simulink model "sim_SS_H2DF_2024a_GRU"  (R2024a)
settings: Solver=FixedStepAuto  StartTime=0.0  StopTime=4899  FixedStep=1  RelTol=1e-3  EnableMultiTasking=on
model workspace (MAT data in the model file):
  enable_IMEP_noise = 100
  enable_IMEP_offset = 1
values from neighbouring files (symbols this model uses):
  C2C_NMPC = init_C2C_NMPC_H2DF(C2C_NMPC.expdata)    [run_SS_H2DF_control.m]
undefined symbols (not defined in the file or in its folder): cost_length, horizon_length, y_ref_buf
libraries: matrix_library x3
(part 2 of 3)

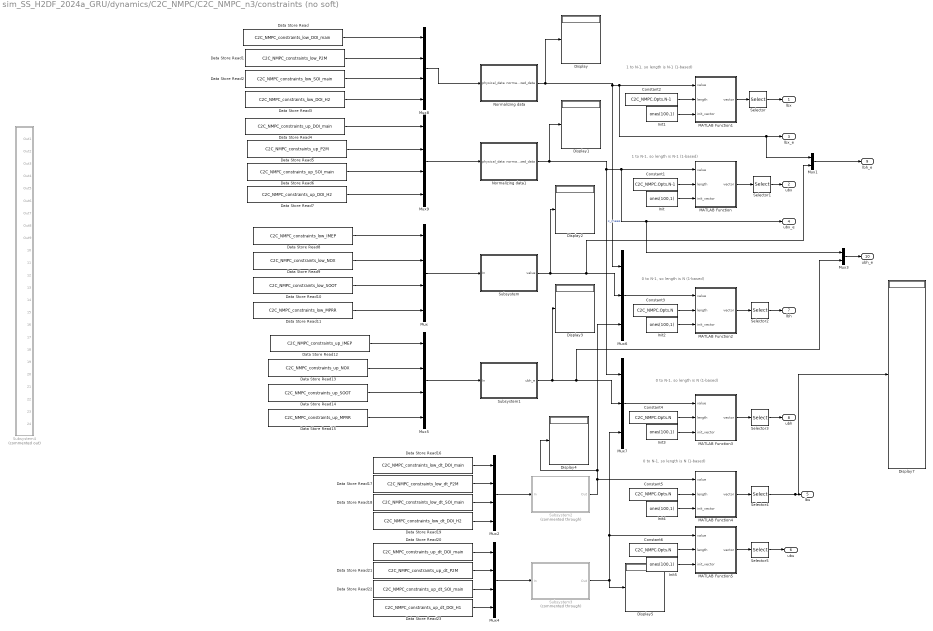
== system sim_SS_H2DF_2024a_GRU/dynamics/C2C_NMPC/C2C_NMPC_n3/constraints (no soft) ==
  note: 1 to N-1, so length is N-1 (1-based)
  note: 1 to N-1, so length is N-1 (1-based)
  note: 0 to N-1, so length is N (1-based)
  note: 0 to N-1, so length is N (1-based)
  note: 0 to N-1, so length is N (1-based)
  Constant1 : Constant  Value=C2C_NMPC.Opts.N-1
  Constant2 : Constant  Value=C2C_NMPC.Opts.N-1
  Constant{3..6} (4 alike) : Constant  Value=C2C_NMPC.Opts.N
  Data Store Read : DataStoreRead  DataStoreName=C2C_NMPC_constraints_low_DOI_main  IndexOptions=Index vector (dialog)  Indices=1  OutputSizes=1
  Data Store Read1 : DataStoreRead  DataStoreName=C2C_NMPC_constraints_low_P2M  IndexOptions=Index vector (dialog)  Indices=1  OutputSizes=1
  Data Store Read10 : DataStoreRead  DataStoreName=C2C_NMPC_constraints_low_SOOT  IndexOptions=Index vector (dialog)  Indices=1  OutputSizes=1
  Data Store Read11 : DataStoreRead  DataStoreName=C2C_NMPC_constraints_low_MPRR  IndexOptions=Index vector (dialog)  Indices=1  OutputSizes=1
  Data Store Read12 : DataStoreRead  DataStoreName=C2C_NMPC_constraints_up_IMEP  IndexOptions=Index vector (dialog)  Indices=1  OutputSizes=1
  Data Store Read13 : DataStoreRead  DataStoreName=C2C_NMPC_constraints_up_NOX  IndexOptions=Index vector (dialog)  Indices=1  OutputSizes=1
  Data Store Read14 : DataStoreRead  DataStoreName=C2C_NMPC_constraints_up_SOOT  IndexOptions=Index vector (dialog)  Indices=1  OutputSizes=1
  Data Store Read15 : DataStoreRead  DataStoreName=C2C_NMPC_constraints_up_MPRR  IndexOptions=Index vector (dialog)  Indices=1  OutputSizes=1
  Data Store Read16 : DataStoreRead  DataStoreName=C2C_NMPC_constraints_low_dt_DOI_main  IndexOptions=Index vector (dialog)  Indices=1  OutputSizes=1
  Data Store Read17 : DataStoreRead  DataStoreName=C2C_NMPC_constraints_low_dt_P2M  IndexOptions=Index vector (dialog)  Indices=1  OutputSizes=1
  Data Store Read18 : DataStoreRead  DataStoreName=C2C_NMPC_constraints_low_dt_SOI_main  IndexOptions=Index vector (dialog)  Indices=1  OutputSizes=1
  Data Store Read19 : DataStoreRead  DataStoreName=C2C_NMPC_constraints_low_dt_DOI_H2  IndexOptions=Index vector (dialog)  Indices=1  OutputSizes=1
  Data Store Read2 : DataStoreRead  DataStoreName=C2C_NMPC_constraints_low_SOI_main  IndexOptions=Index vector (dialog)  Indices=1  OutputSizes=1
  Data Store Read20 : DataStoreRead  DataStoreName=C2C_NMPC_constraints_up_dt_DOI_main  IndexOptions=Index vector (dialog)  Indices=1  OutputSizes=1
  Data Store Read21 : DataStoreRead  DataStoreName=C2C_NMPC_constraints_up_dt_P2M  IndexOptions=Index vector (dialog)  Indices=1  OutputSizes=1
  Data Store Read22 : DataStoreRead  DataStoreName=C2C_NMPC_constraints_up_dt_SOI_main  IndexOptions=Index vector (dialog)  Indices=1  OutputSizes=1
  Data Store Read23 : DataStoreRead  DataStoreName=C2C_NMPC_constraints_up_dt_DOI_H1  IndexOptions=Index vector (dialog)  Indices=1  OutputSizes=1
  Data Store Read3 : DataStoreRead  DataStoreName=C2C_NMPC_constraints_low_DOI_H2  IndexOptions=Index vector (dialog)  Indices=1  OutputSizes=1
  Data Store Read4 : DataStoreRead  DataStoreName=C2C_NMPC_constraints_up_DOI_main  IndexOptions=Index vector (dialog)  Indices=1  OutputSizes=1
  Data Store Read5 : DataStoreRead  DataStoreName=C2C_NMPC_constraints_up_P2M  IndexOptions=Index vector (dialog)  Indices=1  OutputSizes=1
  Data Store Read6 : DataStoreRead  DataStoreName=C2C_NMPC_constraints_up_SOI_main  IndexOptions=Index vector (dialog)  Indices=1  OutputSizes=1
  Data Store Read7 : DataStoreRead  DataStoreName=C2C_NMPC_constraints_up_DOI_H2  IndexOptions=Index vector (dialog)  Indices=1  OutputSizes=1
  Data Store Read8 : DataStoreRead  DataStoreName=C2C_NMPC_constraints_low_IMEP  IndexOptions=Index vector (dialog)  Indices=1  OutputSizes=1
  Data Store Read9 : DataStoreRead  DataStoreName=C2C_NMPC_constraints_low_NOX  IndexOptions=Index vector (dialog)  Indices=1  OutputSizes=1
  Display{,1..5,7} (7 alike) : Display
  Init{,1..5} (6 alike) : Constant  Value=ones(100,1)
  MATLAB Function : MATLAB Function  TreatAsAtomicUnit=on
  MATLAB Function1 : MATLAB Function  TreatAsAtomicUnit=on
  MATLAB Function2 : MATLAB Function  TreatAsAtomicUnit=on
  MATLAB Function3 : MATLAB Function  TreatAsAtomicUnit=on
  MATLAB Function4 : MATLAB Function  TreatAsAtomicUnit=on
  MATLAB Function5 : MATLAB Function  TreatAsAtomicUnit=on
  Mux{,2,4..5,8..9} (6 alike) : Mux
  Mux1 : Mux  Inputs=2
  Mux3 : Mux  Inputs=2
  Mux6 : Mux  Inputs=3
  Mux7 : Mux  Inputs=3
  Normalizing data : Subsystem
  Normalizing data1 : Subsystem
  Selector : Selector  IndexOptions=Index vector (dialog)  Indices=1:((C2C_NMPC.Opts.N-1)*C2C_NMPC.Dims.n_controls)  OutputSizes=1
  Selector1 : Selector  IndexOptions=Index vector (dialog)  Indices=1:((C2C_NMPC.Opts.N-1)*C2C_NMPC.Dims.n_controls)  OutputSizes=1
  Selector2 : Selector  IndexOptions=Index vector (dialog)  Indices=1:((C2C_NMPC.Opts.N)*(C2C_NMPC.Dims.n_outputs + C2C_NMPC.Dims.n_controls +C2C_NMPC.Dims.n_controls))  OutputSizes=1
  Selector3 : Selector  IndexOptions=Index vector (dialog)  Indices=1:((C2C_NMPC.Opts.N)*(C2C_NMPC.Dims.n_outputs + C2C_NMPC.Dims.n_controls +C2C_NMPC.Dims.n_controls))  OutputSizes=1
  Selector4 : Selector  IndexOptions=Index vector (dialog)  Indices=1:((C2C_NMPC.Opts.N)*(C2C_NMPC.Dims.n_controls))  OutputSizes=1
  Selector5 : Selector  IndexOptions=Index vector (dialog)  Indices=1:((C2C_NMPC.Opts.N)*(C2C_NMPC.Dims.n_controls))  OutputSizes=1
  Subsystem : Subsystem
  Subsystem1 : Subsystem
  Subsystem2 : Subsystem  Commented=through
  Subsystem3 : Subsystem  Commented=through
  Subsystem4 : Subsystem  Commented=on
  lbx : Outport
  ubx : Outport  Port=2
  lbx_e : Outport  Port=3
  ubx_e : Outport  Port=4
  lbu : Outport  Port=5
  ubu : Outport  Port=6
  lbh : Outport  Port=7
  ubh : Outport  Port=8
  lbh_e : Outport  Port=9
  ubh_e : Outport  Port=10
  wires:
  Selector4/1 -> lbu/1, Display7/1
  Selector5/1 -> ubu/1
  Constant6/1 -> MATLAB Function5/2(length)
  Init5/1 -> MATLAB Function5/3(init_vector)
  MATLAB Function5/1(vector) -> Selector5/1
  MATLAB Function4/1(vector) -> Selector4/1
  Init4/1 -> MATLAB Function4/3(init_vector)
  Constant5/1 -> MATLAB Function4/2(length)
  Data Store Read23/1 -> Mux4/4
  Data Store Read22/1 -> Mux4/3
  Data Store Read21/1 -> Mux4/2
  Data Store Read20/1 -> Mux4/1
  Data Store Read19/1 -> Mux2/4
  Data Store Read18/1 -> Mux2/3
  Data Store Read17/1 -> Mux2/2
  Data Store Read16/1 -> Mux2/1
  Data Store Read15/1 -> Mux5/4
  Data Store Read14/1 -> Mux5/3
  Data Store Read13/1 -> Mux5/2
  Data Store Read12/1 -> Mux5/1
  Data Store Read11/1 -> Mux/4
  Data Store Read10/1 -> Mux/3
  Data Store Read9/1 -> Mux/2
  Data Store Read8/1 -> Mux/1
  Mux3/1 -> ubh_e/1
  Subsystem1/1(ubh_e) -> Mux7/2, Mux3/2, Display3/1
  Mux1/1 -> lbh_e/1
  Selector3/1 -> ubh/1
  Selector2/1 -> lbh/1
  Selector1/1 -> ubx/1
  Data Store Read7/1 -> Mux9/4
  Normalizing data1/1(normalized_data) -> MATLAB Function/1(value), ubx_e/1, Mux3/1, Mux7/1, Display1/1  "x_meas"
  Mux9/1 -> Normalizing data1/1(physical_data)
  Data Store Read4/1 -> Mux9/1
  Data Store Read5/1 -> Mux9/2
  Data Store Read6/1 -> Mux9/3
  Selector/1 -> lbx/1
  Mux8/1 -> Normalizing data/1(physical_data)
  Data Store Read/1 -> Mux8/1
  Data Store Read1/1 -> Mux8/2
  Data Store Read2/1 -> Mux8/3
  Data Store Read3/1 -> Mux8/4
  Constant4/1 -> MATLAB Function3/2(length)
  Init3/1 -> MATLAB Function3/3(init_vector)
  Mux7/1 -> MATLAB Function3/1(value)
  MATLAB Function3/1(vector) -> Selector3/1
  Subsystem2/1(Out) -> Mux6/3, Display4/1, MATLAB Function4/1(value)
  Subsystem/1(value) -> Mux6/2, Mux1/2, Display2/1
  Normalizing data/1(normalized_data) -> Display/1, MATLAB Function1/1(value), lbx_e/1, Mux1/1, Mux6/1
  Mux6/1 -> MATLAB Function2/1(value)
  Subsystem3/1(Out) -> Display5/1, Mux7/3, MATLAB Function5/1(value)
  Init2/1 -> MATLAB Function2/3(init_vector)
  Constant3/1 -> MATLAB Function2/2(length)
  MATLAB Function2/1(vector) -> Selector2/1
  Init1/1 -> MATLAB Function1/3(init_vector)
  Constant2/1 -> MATLAB Function1/2(length)
  MATLAB Function1/1(vector) -> Selector/1
  MATLAB Function/1(vector) -> Selector1/1
  Constant1/1 -> MATLAB Function/2(length)
  Init/1 -> MATLAB Function/3(init_vector)
  Mux4/1 -> Subsystem3/1(In)
  Mux2/1 -> Subsystem2/1(In)
  Mux5/1 -> Subsystem1/1(In)
  Mux/1 -> Subsystem/1(In)

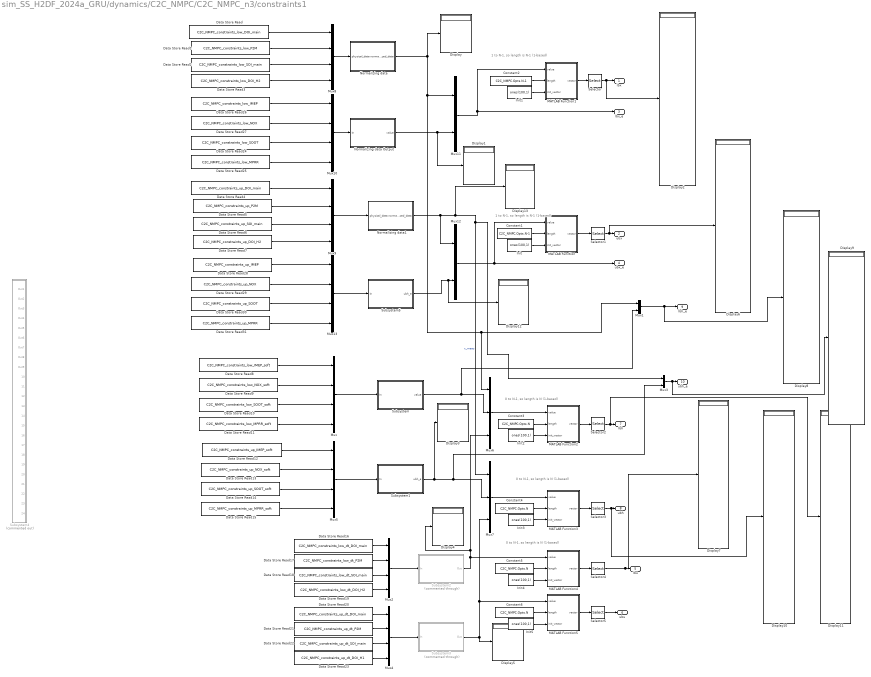
== system sim_SS_H2DF_2024a_GRU/dynamics/C2C_NMPC/C2C_NMPC_n3/constraints1 ==
  note: 0 to N-1, so length is N (1-based)
  note: 0 to N-1, so length is N (1-based)
  note: 0 to N-1, so length is N (1-based)
  note: 1 to N-1, so length is N-1 (1-based)
  note: 1 to N-1, so length is N-1 (1-based)
  Constant1 : Constant  Value=C2C_NMPC.Opts.N-1
  Constant2 : Constant  Value=C2C_NMPC.Opts.N-1
  Constant{3..6} (4 alike) : Constant  Value=C2C_NMPC.Opts.N
  Data Store Read : DataStoreRead  DataStoreName=C2C_NMPC_constraints_low_DOI_main  IndexOptions=Index vector (dialog)  Indices=1  OutputSizes=1
  Data Store Read1 : DataStoreRead  DataStoreName=C2C_NMPC_constraints_low_P2M  IndexOptions=Index vector (dialog)  Indices=1  OutputSizes=1
  Data Store Read10 : DataStoreRead  DataStoreName=C2C_NMPC_constraints_low_SOOT_soft  IndexOptions=Index vector (dialog)  Indices=1  OutputSizes=1
  Data Store Read11 : DataStoreRead  DataStoreName=C2C_NMPC_constraints_low_MPRR_soft  IndexOptions=Index vector (dialog)  Indices=1  OutputSizes=1
  Data Store Read12 : DataStoreRead  DataStoreName=C2C_NMPC_constraints_up_IMEP_soft  IndexOptions=Index vector (dialog)  Indices=1  OutputSizes=1
  Data Store Read13 : DataStoreRead  DataStoreName=C2C_NMPC_constraints_up_NOX_soft  IndexOptions=Index vector (dialog)  Indices=1  OutputSizes=1
  Data Store Read14 : DataStoreRead  DataStoreName=C2C_NMPC_constraints_up_SOOT_soft  IndexOptions=Index vector (dialog)  Indices=1  OutputSizes=1
  Data Store Read15 : DataStoreRead  DataStoreName=C2C_NMPC_constraints_up_MPRR_soft  IndexOptions=Index vector (dialog)  Indices=1  OutputSizes=1
  Data Store Read16 : DataStoreRead  DataStoreName=C2C_NMPC_constraints_low_dt_DOI_main  IndexOptions=Index vector (dialog)  Indices=1  OutputSizes=1
  Data Store Read17 : DataStoreRead  DataStoreName=C2C_NMPC_constraints_low_dt_P2M  IndexOptions=Index vector (dialog)  Indices=1  OutputSizes=1
  Data Store Read18 : DataStoreRead  DataStoreName=C2C_NMPC_constraints_low_dt_SOI_main  IndexOptions=Index vector (dialog)  Indices=1  OutputSizes=1
  Data Store Read19 : DataStoreRead  DataStoreName=C2C_NMPC_constraints_low_dt_DOI_H2  IndexOptions=Index vector (dialog)  Indices=1  OutputSizes=1
  Data Store Read2 : DataStoreRead  DataStoreName=C2C_NMPC_constraints_low_SOI_main  IndexOptions=Index vector (dialog)  Indices=1  OutputSizes=1
  Data Store Read20 : DataStoreRead  DataStoreName=C2C_NMPC_constraints_up_dt_DOI_main  IndexOptions=Index vector (dialog)  Indices=1  OutputSizes=1
  Data Store Read21 : DataStoreRead  DataStoreName=C2C_NMPC_constraints_up_dt_P2M  IndexOptions=Index vector (dialog)  Indices=1  OutputSizes=1
  Data Store Read22 : DataStoreRead  DataStoreName=C2C_NMPC_constraints_up_dt_SOI_main  IndexOptions=Index vector (dialog)  Indices=1  OutputSizes=1
  Data Store Read23 : DataStoreRead  DataStoreName=C2C_NMPC_constraints_up_dt_DOI_H1  IndexOptions=Index vector (dialog)  Indices=1  OutputSizes=1
  Data Store Read24 : DataStoreRead  DataStoreName=C2C_NMPC_constraints_low_SOOT  IndexOptions=Index vector (dialog)  Indices=1  OutputSizes=1
  Data Store Read25 : DataStoreRead  DataStoreName=C2C_NMPC_constraints_low_MPRR  IndexOptions=Index vector (dialog)  Indices=1  OutputSizes=1
  Data Store Read26 : DataStoreRead  DataStoreName=C2C_NMPC_constraints_low_IMEP  IndexOptions=Index vector (dialog)  Indices=1  OutputSizes=1
  Data Store Read27 : DataStoreRead  DataStoreName=C2C_NMPC_constraints_low_NOX  IndexOptions=Index vector (dialog)  Indices=1  OutputSizes=1
  Data Store Read28 : DataStoreRead  DataStoreName=C2C_NMPC_constraints_up_IMEP  IndexOptions=Index vector (dialog)  Indices=1  OutputSizes=1
  Data Store Read29 : DataStoreRead  DataStoreName=C2C_NMPC_constraints_up_NOX  IndexOptions=Index vector (dialog)  Indices=1  OutputSizes=1
  Data Store Read3 : DataStoreRead  DataStoreName=C2C_NMPC_constraints_low_DOI_H2  IndexOptions=Index vector (dialog)  Indices=1  OutputSizes=1
  Data Store Read30 : DataStoreRead  DataStoreName=C2C_NMPC_constraints_up_SOOT  IndexOptions=Index vector (dialog)  Indices=1  OutputSizes=1
  Data Store Read31 : DataStoreRead  DataStoreName=C2C_NMPC_constraints_up_MPRR  IndexOptions=Index vector (dialog)  Indices=1  OutputSizes=1
  Data Store Read4 : DataStoreRead  DataStoreName=C2C_NMPC_constraints_up_DOI_main  IndexOptions=Index vector (dialog)  Indices=1  OutputSizes=1
  Data Store Read5 : DataStoreRead  DataStoreName=C2C_NMPC_constraints_up_P2M  IndexOptions=Index vector (dialog)  Indices=1  OutputSizes=1
  Data Store Read6 : DataStoreRead  DataStoreName=C2C_NMPC_constraints_up_SOI_main  IndexOptions=Index vector (dialog)  Indices=1  OutputSizes=1
  Data Store Read7 : DataStoreRead  DataStoreName=C2C_NMPC_constraints_up_DOI_H2  IndexOptions=Index vector (dialog)  Indices=1  OutputSizes=1
  Data Store Read8 : DataStoreRead  DataStoreName=C2C_NMPC_constraints_low_IMEP_soft  IndexOptions=Index vector (dialog)  Indices=1  OutputSizes=1
  Data Store Read9 : DataStoreRead  DataStoreName=C2C_NMPC_constraints_low_NOX_soft  IndexOptions=Index vector (dialog)  Indices=1  OutputSizes=1
  Display{,1..13} (14 alike) : Display
  Init{,1..5} (6 alike) : Constant  Value=ones(100,1)
  MATLAB Function : MATLAB Function  TreatAsAtomicUnit=on
  MATLAB Function1 : MATLAB Function  TreatAsAtomicUnit=on
  MATLAB Function2 : MATLAB Function  TreatAsAtomicUnit=on
  MATLAB Function3 : MATLAB Function  TreatAsAtomicUnit=on
  MATLAB Function4 : MATLAB Function  TreatAsAtomicUnit=on
  MATLAB Function5 : MATLAB Function  TreatAsAtomicUnit=on
  Mux{,2,4..5,8..10,13} (8 alike) : Mux
  Mux{1,3,11..12} (4 alike) : Mux  Inputs=2
  Mux6 : Mux  Inputs=3
  Mux7 : Mux  Inputs=3
  Normalizing data : Subsystem
  Normalizing data Output : Subsystem
  Normalizing data1 : Subsystem
  Selector : Selector  IndexOptions=Index vector (dialog)  Indices=1:((C2C_NMPC.Opts.N-1)*(C2C_NMPC.Dims.n_controls+C2C_NMPC.Dims.n_outputs))  OutputSizes=1
  Selector1 : Selector  IndexOptions=Index vector (dialog)  Indices=1:((C2C_NMPC.Opts.N-1)*(C2C_NMPC.Dims.n_controls+C2C_NMPC.Dims.n_outputs))  OutputSizes=1
  Selector2 : Selector  IndexOptions=Index vector (dialog)  Indices=1:((C2C_NMPC.Opts.N-1)*(C2C_NMPC.Dims.n_outputs + C2C_NMPC.Dims.n_controls +C2C_NMPC.Dims.n_controls))  OutputSizes=1
  Selector3 : Selector  IndexOptions=Index vector (dialog)  Indices=1:((C2C_NMPC.Opts.N-1)*(C2C_NMPC.Dims.n_outputs + C2C_NMPC.Dims.n_controls +C2C_NMPC.Dims.n_controls))  OutputSizes=1
  Selector4 : Selector  IndexOptions=Index vector (dialog)  Indices=1:((C2C_NMPC.Opts.N)*(C2C_NMPC.Dims.n_controls))  OutputSizes=1
  Selector5 : Selector  IndexOptions=Index vector (dialog)  Indices=1:((C2C_NMPC.Opts.N)*(C2C_NMPC.Dims.n_controls))  OutputSizes=1
  Subsystem : Subsystem
  Subsystem1 : Subsystem
  Subsystem2 : Subsystem  Commented=through
  Subsystem3 : Subsystem  Commented=through
  Subsystem4 : Subsystem  Commented=on
  Subsystem5 : Subsystem
  lbx : Outport
  ubx : Outport  Port=2
  lbx_e : Outport  Port=3
  ubx_e : Outport  Port=4
  lbu : Outport  Port=5
  ubu : Outport  Port=6
  lbh : Outport  Port=7
  ubh : Outport  Port=8
  lbh_e : Outport  Port=9
  ubh_e : Outport  Port=10
  wires:
  Mux/1 -> Subsystem/1(In)
  Mux5/1 -> Subsystem1/1(In)
  Mux2/1 -> Subsystem2/1(In)
  Mux4/1 -> Subsystem3/1(In)
  Init/1 -> MATLAB Function/3(init_vector)
  Constant1/1 -> MATLAB Function/2(length)
  MATLAB Function/1(vector) -> Selector1/1
  MATLAB Function1/1(vector) -> Selector/1
  Constant2/1 -> MATLAB Function1/2(length)
  Init1/1 -> MATLAB Function1/3(init_vector)
  MATLAB Function2/1(vector) -> Selector2/1
  Constant3/1 -> MATLAB Function2/2(length)
  Init2/1 -> MATLAB Function2/3(init_vector)
  Subsystem3/1(Out) -> MATLAB Function5/1(value), Mux7/3, Display5/1
  Mux6/1 -> MATLAB Function2/1(value)
  Subsystem/1(value) -> Mux1/2, Mux6/2
  Subsystem2/1(Out) -> MATLAB Function4/1(value), Display4/1, Mux6/3
  MATLAB Function3/1(vector) -> Selector3/1
  Mux7/1 -> MATLAB Function3/1(value)
  Init3/1 -> MATLAB Function3/3(init_vector)
  Constant4/1 -> MATLAB Function3/2(length)
  Data Store Read3/1 -> Mux8/4
  Data Store Read2/1 -> Mux8/3
  Data Store Read1/1 -> Mux8/2
  Data Store Read/1 -> Mux8/1
  Mux8/1 -> Normalizing data/1(physical_data)
  Selector/1 -> Display2/1, lbx/1
  Data Store Read6/1 -> Mux9/3
  Data Store Read5/1 -> Mux9/2
  Data Store Read4/1 -> Mux9/1
  Mux9/1 -> Normalizing data1/1(physical_data)
  Normalizing data1/1(normalized_data) -> Mux12/1, Display13/1, Mux7/1, Mux3/1  "x_meas"
  Data Store Read7/1 -> Mux9/4
  Selector1/1 -> Display6/1, ubx/1
  Selector2/1 -> Display11/1, lbh/1
  Selector3/1 -> Display10/1, ubh/1
  Mux1/1 -> Display8/1, lbh_e/1
  Subsystem1/1(ubh_e) -> Display3/1, Mux3/2, Mux7/2
  Mux3/1 -> Display9/1, ubh_e/1
  Data Store Read8/1 -> Mux/1
  Data Store Read9/1 -> Mux/2
  Data Store Read10/1 -> Mux/3
  Data Store Read11/1 -> Mux/4
  Data Store Read12/1 -> Mux5/1
  Data Store Read13/1 -> Mux5/2
  Data Store Read14/1 -> Mux5/3
  Data Store Read15/1 -> Mux5/4
  Data Store Read16/1 -> Mux2/1
  Data Store Read17/1 -> Mux2/2
  Data Store Read18/1 -> Mux2/3
  Data Store Read19/1 -> Mux2/4
  Data Store Read20/1 -> Mux4/1
  Data Store Read21/1 -> Mux4/2
  Data Store Read22/1 -> Mux4/3
  Data Store Read23/1 -> Mux4/4
  Constant5/1 -> MATLAB Function4/2(length)
  Init4/1 -> MATLAB Function4/3(init_vector)
  MATLAB Function4/1(vector) -> Selector4/1
  MATLAB Function5/1(vector) -> Selector5/1
  Init5/1 -> MATLAB Function5/3(init_vector)
  Constant6/1 -> MATLAB Function5/2(length)
  Selector5/1 -> ubu/1
  Selector4/1 -> Display7/1, lbu/1
  Data Store Read27/1 -> Mux10/2
  Data Store Read26/1 -> Mux10/1
  Data Store Read24/1 -> Mux10/3
  Data Store Read25/1 -> Mux10/4
  Mux10/1 -> Normalizing data Output/1(In)
  Mux11/1 -> lbx_e/1, MATLAB Function1/1(value)
  Normalizing data Output/1(value) -> Display1/1, Mux11/2
  Mux12/1 -> MATLAB Function/1(value), ubx_e/1
  Mux13/1 -> Subsystem5/1(In)
  Data Store Read30/1 -> Mux13/3
  Data Store Read29/1 -> Mux13/2
  Data Store Read28/1 -> Mux13/1
  Subsystem5/1(ubh_e) -> Display12/1, Mux12/2
  Data Store Read31/1 -> Mux13/4
  Normalizing data/1(normalized_data) -> Mux6/1, Mux1/1, Mux11/1, Display/1

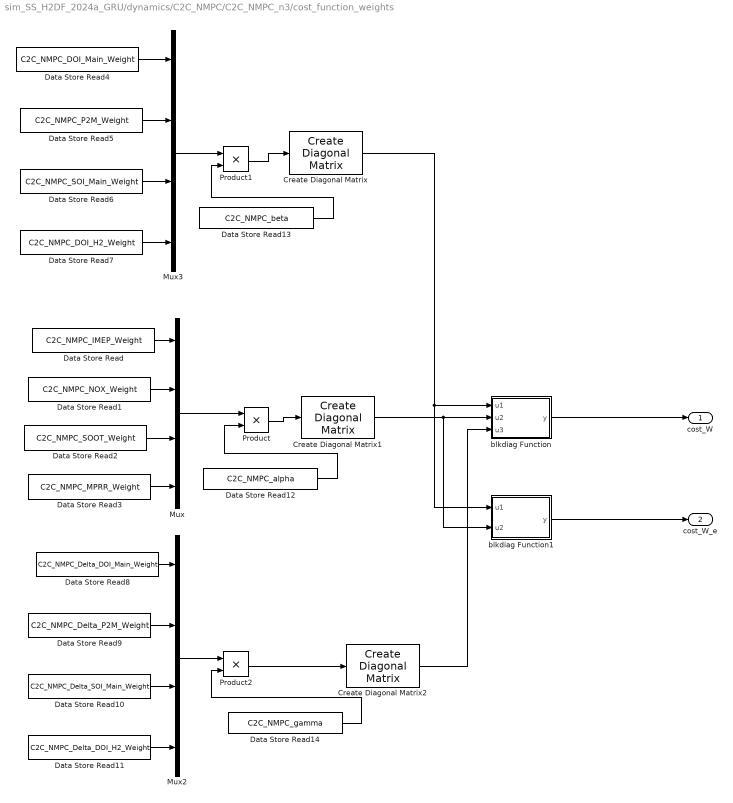
== system sim_SS_H2DF_2024a_GRU/dynamics/C2C_NMPC/C2C_NMPC_n3/cost_function_weights ==
  Create Diagonal Matrix : matrix_library/Create Diagonal Matrix
  Create Diagonal Matrix1 : matrix_library/Create Diagonal Matrix
  Create Diagonal Matrix2 : matrix_library/Create Diagonal Matrix
  Data Store Read : DataStoreRead  DataStoreName=C2C_NMPC_IMEP_Weight  IndexOptions=Index vector (dialog)  Indices=1  OutputSizes=1
  Data Store Read1 : DataStoreRead  DataStoreName=C2C_NMPC_NOX_Weight  IndexOptions=Index vector (dialog)  Indices=1  OutputSizes=1
  Data Store Read10 : DataStoreRead  DataStoreName=C2C_NMPC_Delta_SOI_Main_Weight  IndexOptions=Index vector (dialog)  Indices=1  OutputSizes=1
  Data Store Read11 : DataStoreRead  DataStoreName=C2C_NMPC_Delta_DOI_H2_Weight  IndexOptions=Index vector (dialog)  Indices=1  OutputSizes=1
  Data Store Read12 : DataStoreRead  DataStoreName=C2C_NMPC_alpha  IndexOptions=Index vector (dialog)  Indices=1  OutputSizes=1
  Data Store Read13 : DataStoreRead  DataStoreName=C2C_NMPC_beta  IndexOptions=Index vector (dialog)  Indices=1  OutputSizes=1
  Data Store Read14 : DataStoreRead  DataStoreName=C2C_NMPC_gamma  IndexOptions=Index vector (dialog)  Indices=1  OutputSizes=1
  Data Store Read2 : DataStoreRead  DataStoreName=C2C_NMPC_SOOT_Weight  IndexOptions=Index vector (dialog)  Indices=1  OutputSizes=1
  Data Store Read3 : DataStoreRead  DataStoreName=C2C_NMPC_MPRR_Weight  IndexOptions=Index vector (dialog)  Indices=1  OutputSizes=1
  Data Store Read4 : DataStoreRead  DataStoreName=C2C_NMPC_DOI_Main_Weight  IndexOptions=Index vector (dialog)  Indices=1  OutputSizes=1
  Data Store Read5 : DataStoreRead  DataStoreName=C2C_NMPC_P2M_Weight  IndexOptions=Index vector (dialog)  Indices=1  OutputSizes=1
  Data Store Read6 : DataStoreRead  DataStoreName=C2C_NMPC_SOI_Main_Weight  IndexOptions=Index vector (dialog)  Indices=1  OutputSizes=1
  Data Store Read7 : DataStoreRead  DataStoreName=C2C_NMPC_DOI_H2_Weight  IndexOptions=Index vector (dialog)  Indices=1  OutputSizes=1
  Data Store Read8 : DataStoreRead  DataStoreName=C2C_NMPC_Delta_DOI_Main_Weight  IndexOptions=Index vector (dialog)  Indices=1  OutputSizes=1
  Data Store Read9 : DataStoreRead  DataStoreName=C2C_NMPC_Delta_P2M_Weight  IndexOptions=Index vector (dialog)  Indices=1  OutputSizes=1
  Mux : Mux
  Mux2 : Mux
  Mux3 : Mux
  Product : Product
  Product1 : Product
  Product2 : Product
  blkdiag Function : MATLAB Function  TreatAsAtomicUnit=on
  blkdiag Function1 : MATLAB Function  TreatAsAtomicUnit=on
  cost_W : Outport
  cost_W_e : Outport  Port=2
  wires:
  blkdiag Function1/1(y) -> cost_W_e/1
  Mux2/1 -> Product2/1
  Data Store Read14/1 -> Product2/2
  Data Store Read13/1 -> Product1/2
  Data Store Read12/1 -> Product/2
  Data Store Read11/1 -> Mux2/4
  Data Store Read10/1 -> Mux2/3
  Data Store Read9/1 -> Mux2/2
  Data Store Read8/1 -> Mux2/1
  Create Diagonal Matrix/1 -> blkdiag Function/1(u1), blkdiag Function1/1(u1)
  Data Store Read2/1 -> Mux/3
  Data Store Read3/1 -> Mux/4
  Data Store Read/1 -> Mux/1
  Data Store Read1/1 -> Mux/2
  Mux/1 -> Product/1
  Product/1 -> Create Diagonal Matrix1/1
  Product1/1 -> Create Diagonal Matrix/1
  Mux3/1 -> Product1/1
  Data Store Read5/1 -> Mux3/2
  Data Store Read6/1 -> Mux3/3
  Data Store Read4/1 -> Mux3/1
  Data Store Read7/1 -> Mux3/4
  Create Diagonal Matrix1/1 -> blkdiag Function/2(u2), blkdiag Function1/2(u2)
  Product2/1 -> Create Diagonal Matrix2/1
  Create Diagonal Matrix2/1 -> blkdiag Function/3(u3)
  blkdiag Function/1(y) -> cost_W/1

== system sim_SS_H2DF_2024a_GRU/dynamics/C2C_NMPC/C2C_NMPC_n3/constraints (no soft)/Normalizing data ==
  physical_data : Inport
  Constant1 : Constant  Value=C2C_NMPC.Normalization.controls.mean(2)
  Constant2 : Constant  Value=C2C_NMPC.Normalization.controls.mean(3)
  Constant3 : Constant  Value=C2C_NMPC.Normalization.controls.mean(1)
  Constant4 : Constant  Value=C2C_NMPC.Normalization.controls.mean(4)
  Gain1 : Gain  Gain=1/C2C_NMPC.Normalization.controls.std(2)
  Gain2 : Gain  Gain=1/C2C_NMPC.Normalization.controls.std(3)
  Gain3 : Gain  Gain=1/C2C_NMPC.Normalization.controls.std(4)
  Gain4 : Gain  Gain=1/C2C_NMPC.Normalization.controls.std(1)
  Mux : Mux
  Selector : Selector  IndexOptions=Index vector (dialog)  Indices=[2]  OutputSizes=1
  Selector1 : Selector  IndexOptions=Index vector (dialog)  Indices=[1]  OutputSizes=1
  Selector2 : Selector  IndexOptions=Index vector (dialog)  Indices=[3]  OutputSizes=1
  Selector3 : Selector  IndexOptions=Index vector (dialog)  Indices=[4]  OutputSizes=1
  Sum{1..4} (4 alike) : Sum  Inputs=|+-
  normalized_data : Outport
  wires:
  physical_data/1 -> Selector2/1, Selector3/1, Selector/1, Selector1/1
  Mux/1 -> normalized_data/1
  Gain3/1 -> Mux/4
  Gain2/1 -> Mux/3
  Gain1/1 -> Mux/2
  Gain4/1 -> Mux/1
  Selector1/1 -> Sum4/1
  Selector3/1 -> Sum1/1
  Constant4/1 -> Sum1/2
  Sum1/1 -> Gain3/1
  Sum2/1 -> Gain1/1
  Constant1/1 -> Sum2/2
  Selector/1 -> Sum2/1
  Sum3/1 -> Gain2/1
  Sum4/1 -> Gain4/1
  Constant2/1 -> Sum3/2
  Selector2/1 -> Sum3/1
  Constant3/1 -> Sum4/2

== system sim_SS_H2DF_2024a_GRU/dynamics/C2C_NMPC/C2C_NMPC_n3/constraints (no soft)/Normalizing data1 ==
  physical_data : Inport
  Constant1 : Constant  Value=C2C_NMPC.Normalization.controls.mean(2)
  Constant2 : Constant  Value=C2C_NMPC.Normalization.controls.mean(3)
  Constant3 : Constant  Value=C2C_NMPC.Normalization.controls.mean(1)
  Constant4 : Constant  Value=C2C_NMPC.Normalization.controls.mean(4)
  Gain1 : Gain  Gain=1/C2C_NMPC.Normalization.controls.std(2)
  Gain2 : Gain  Gain=1/C2C_NMPC.Normalization.controls.std(3)
  Gain3 : Gain  Gain=1/C2C_NMPC.Normalization.controls.std(4)
  Gain4 : Gain  Gain=1/C2C_NMPC.Normalization.controls.std(1)
  Mux : Mux
  Selector : Selector  IndexOptions=Index vector (dialog)  Indices=[2]  OutputSizes=1
  Selector1 : Selector  IndexOptions=Index vector (dialog)  Indices=[1]  OutputSizes=1
  Selector2 : Selector  IndexOptions=Index vector (dialog)  Indices=[3]  OutputSizes=1
  Selector3 : Selector  IndexOptions=Index vector (dialog)  Indices=[4]  OutputSizes=1
  Sum{1..4} (4 alike) : Sum  Inputs=|+-
  normalized_data : Outport
  wires:
  physical_data/1 -> Selector2/1, Selector3/1, Selector/1, Selector1/1
  Mux/1 -> normalized_data/1
  Gain3/1 -> Mux/4
  Gain2/1 -> Mux/3
  Gain1/1 -> Mux/2
  Gain4/1 -> Mux/1
  Selector1/1 -> Sum4/1
  Selector3/1 -> Sum1/1
  Constant4/1 -> Sum1/2
  Sum1/1 -> Gain3/1
  Sum2/1 -> Gain1/1
  Constant1/1 -> Sum2/2
  Selector/1 -> Sum2/1
  Sum3/1 -> Gain2/1
  Sum4/1 -> Gain4/1
  Constant2/1 -> Sum3/2
  Selector2/1 -> Sum3/1
  Constant3/1 -> Sum4/2

== system sim_SS_H2DF_2024a_GRU/dynamics/C2C_NMPC/C2C_NMPC_n3/constraints (no soft)/Subsystem ==
  In : Inport
  Constant : Constant  Value=C2C_NMPC.Normalization.outputs.mean(1)
  Constant1 : Constant  Value=C2C_NMPC.Normalization.outputs.mean(2)
  Constant2 : Constant  Value=C2C_NMPC.Normalization.outputs.mean(3)
  Constant3 : Constant  Value=C2C_NMPC.Normalization.outputs.mean(4)
  Demux : Demux
  Gain : Gain  Gain=1/C2C_NMPC.Normalization.outputs.std(1)
  Gain1 : Gain  Gain=1/C2C_NMPC.Normalization.outputs.std(2)
  Gain2 : Gain  Gain=1/C2C_NMPC.Normalization.outputs.std(3)
  Gain3 : Gain  Gain=1/C2C_NMPC.Normalization.outputs.std(4)
  Mux : Mux
  Sum{1..3,5} (4 alike) : Sum  Inputs=|+-
  value : Outport
  wires:
  Mux/1 -> value/1
  In/1 -> Demux/1
  Demux/4 -> Sum3/1
  Demux/2 -> Sum1/1
  Gain1/1 -> Mux/2
  Gain3/1 -> Mux/4
  Gain2/1 -> Mux/3
  Demux/1 -> Sum5/1
  Sum5/1 -> Gain/1
  Constant3/1 -> Sum3/2
  Sum3/1 -> Gain3/1
  Gain/1 -> Mux/1
  Constant2/1 -> Sum2/2
  Sum2/1 -> Gain2/1
  Demux/3 -> Sum2/1
  Sum1/1 -> Gain1/1
  Constant1/1 -> Sum1/2
  Constant/1 -> Sum5/2

== system sim_SS_H2DF_2024a_GRU/dynamics/C2C_NMPC/C2C_NMPC_n3/constraints (no soft)/Subsystem1 ==
  In : Inport
  Constant : Constant  Value=C2C_NMPC.Normalization.outputs.mean(1)
  Constant1 : Constant  Value=C2C_NMPC.Normalization.outputs.mean(2)
  Constant2 : Constant  Value=C2C_NMPC.Normalization.outputs.mean(3)
  Constant3 : Constant  Value=C2C_NMPC.Normalization.outputs.mean(4)
  Demux : Demux
  Gain : Gain  Gain=1/C2C_NMPC.Normalization.outputs.std(1)
  Gain1 : Gain  Gain=1/C2C_NMPC.Normalization.outputs.std(2)
  Gain2 : Gain  Gain=1/C2C_NMPC.Normalization.outputs.std(3)
  Gain3 : Gain  Gain=1/C2C_NMPC.Normalization.outputs.std(4)
  Mux : Mux
  Sum{1..3,5} (4 alike) : Sum  Inputs=|+-
  ubh_e : Outport
  wires:
  Constant/1 -> Sum5/2
  Constant1/1 -> Sum1/2
  Sum1/1 -> Gain1/1
  Demux/3 -> Sum2/1
  Sum2/1 -> Gain2/1
  Constant2/1 -> Sum2/2
  Gain/1 -> Mux/1
  Sum3/1 -> Gain3/1
  Constant3/1 -> Sum3/2
  Sum5/1 -> Gain/1
  Demux/1 -> Sum5/1
  Gain2/1 -> Mux/3
  Gain3/1 -> Mux/4
  Gain1/1 -> Mux/2
  Demux/2 -> Sum1/1
  Demux/4 -> Sum3/1
  In/1 -> Demux/1
  Mux/1 -> ubh_e/1

== system sim_SS_H2DF_2024a_GRU/dynamics/C2C_NMPC/C2C_NMPC_n3/constraints (no soft)/Subsystem2 ==
  In : Inport
  Demux : Demux
  Gain : Gain  Gain=1/C2C_NMPC.Normalization.controls.std(1)
  Gain1 : Gain  Gain=1/C2C_NMPC.Normalization.controls.std(2)
  Gain2 : Gain  Gain=1/C2C_NMPC.Normalization.controls.std(3)
  Gain3 : Gain  Gain=1/C2C_NMPC.Normalization.controls.std(4)
  Mux : Mux
  Out : Outport
  wires:
  Gain3/1 -> Mux/4
  Demux/4 -> Gain3/1
  Demux/3 -> Gain2/1
  Demux/2 -> Gain1/1
  Demux/1 -> Gain/1
  Mux/1 -> Out/1
  In/1 -> Demux/1
  Gain1/1 -> Mux/2
  Gain2/1 -> Mux/3
  Gain/1 -> Mux/1

== system sim_SS_H2DF_2024a_GRU/dynamics/C2C_NMPC/C2C_NMPC_n3/constraints (no soft)/Subsystem3 ==
  In : Inport
  Demux : Demux
  Gain : Gain  Gain=1/C2C_NMPC.Normalization.controls.std(1)
  Gain1 : Gain  Gain=1/C2C_NMPC.Normalization.controls.std(2)
  Gain2 : Gain  Gain=1/C2C_NMPC.Normalization.controls.std(3)
  Gain3 : Gain  Gain=1/C2C_NMPC.Normalization.controls.std(4)
  Mux : Mux
  Out : Outport
  wires:
  Gain3/1 -> Mux/4
  Demux/4 -> Gain3/1
  Demux/3 -> Gain2/1
  Demux/2 -> Gain1/1
  Demux/1 -> Gain/1
  Mux/1 -> Out/1
  In/1 -> Demux/1
  Gain1/1 -> Mux/2
  Gain2/1 -> Mux/3
  Gain/1 -> Mux/1

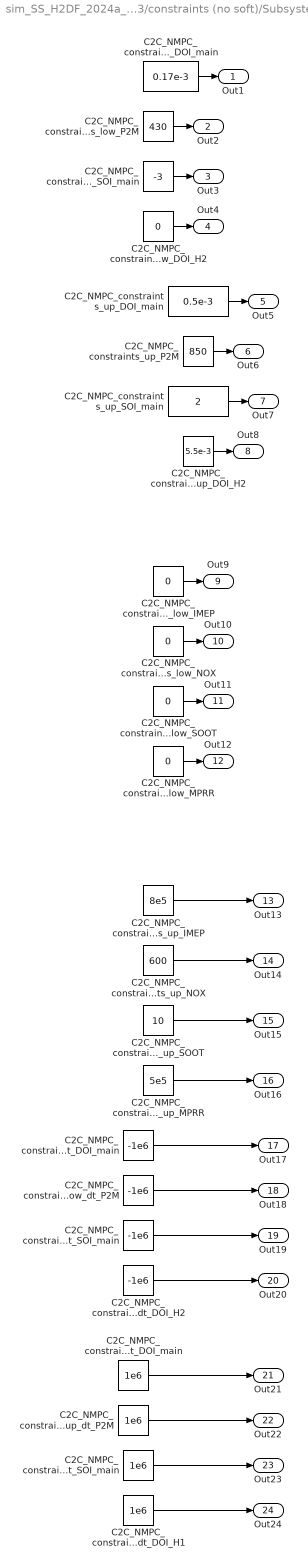
== system sim_SS_H2DF_2024a_GRU/dynamics/C2C_NMPC/C2C_NMPC_n3/constraints (no soft)/Subsystem4 ==
  C2C_NMPC_constraints_low_DOI_H2 : Constant  Value=0
  C2C_NMPC_constraints_low_DOI_main : Constant  Value=0.17e-3
  C2C_NMPC_constraints_low_IMEP : Constant  Value=0
  C2C_NMPC_constraints_low_MPRR : Constant  Value=0
  C2C_NMPC_constraints_low_NOX : Constant  Value=0
  C2C_NMPC_constraints_low_P2M : Constant  Value=430
  C2C_NMPC_constraints_low_SOI_main : Constant  Value=-3
  C2C_NMPC_constraints_low_SOOT : Constant  Value=0
  C2C_NMPC_constraints_low_dt_DOI_H2 : Constant  Value=-1e6
  C2C_NMPC_constraints_low_dt_DOI_main : Constant  Value=-1e6
  C2C_NMPC_constraints_low_dt_P2M : Constant  Value=-1e6
  C2C_NMPC_constraints_low_dt_SOI_main : Constant  Value=-1e6
  C2C_NMPC_constraints_up_DOI_H2 : Constant  Value=5.5e-3
  C2C_NMPC_constraints_up_DOI_main : Constant  Value=0.5e-3
  C2C_NMPC_constraints_up_IMEP : Constant  Value=8e5
  C2C_NMPC_constraints_up_MPRR : Constant  Value=5e5
  C2C_NMPC_constraints_up_NOX : Constant  Value=600
  C2C_NMPC_constraints_up_P2M : Constant  Value=850
  C2C_NMPC_constraints_up_SOI_main : Constant  Value=2
  C2C_NMPC_constraints_up_SOOT : Constant  Value=10
  C2C_NMPC_constraints_up_dt_DOI_H1 : Constant  Value=1e6
  C2C_NMPC_constraints_up_dt_DOI_main : Constant  Value=1e6
  C2C_NMPC_constraints_up_dt_P2M : Constant  Value=1e6
  C2C_NMPC_constraints_up_dt_SOI_main : Constant  Value=1e6
  Out1 : Outport
  Out2 : Outport  Port=2
  Out3 : Outport  Port=3
  Out4 : Outport  Port=4
  Out5 : Outport  Port=5
  Out6 : Outport  Port=6
  Out7 : Outport  Port=7
  Out8 : Outport  Port=8
  Out9 : Outport  Port=9
  Out10 : Outport  Port=10
  Out11 : Outport  Port=11
  Out12 : Outport  Port=12
  Out13 : Outport  Port=13
  Out14 : Outport  Port=14
  Out15 : Outport  Port=15
  Out16 : Outport  Port=16
  Out17 : Outport  Port=17
  Out18 : Outport  Port=18
  Out19 : Outport  Port=19
  Out20 : Outport  Port=20
  Out21 : Outport  Port=21
  Out22 : Outport  Port=22
  Out23 : Outport  Port=23
  Out24 : Outport  Port=24
  wires:
  C2C_NMPC_constraints_low_NOX/1 -> Out10/1
  C2C_NMPC_constraints_low_IMEP/1 -> Out9/1
  C2C_NMPC_constraints_up_DOI_main/1 -> Out5/1
  C2C_NMPC_constraints_up_SOI_main/1 -> Out7/1
  C2C_NMPC_constraints_low_MPRR/1 -> Out12/1
  C2C_NMPC_constraints_low_DOI_main/1 -> Out1/1
  C2C_NMPC_constraints_low_P2M/1 -> Out2/1
  C2C_NMPC_constraints_up_P2M/1 -> Out6/1
  C2C_NMPC_constraints_low_DOI_H2/1 -> Out4/1
  C2C_NMPC_constraints_low_SOOT/1 -> Out11/1
  C2C_NMPC_constraints_up_dt_DOI_main/1 -> Out21/1
  C2C_NMPC_constraints_low_SOI_main/1 -> Out3/1
  C2C_NMPC_constraints_up_dt_P2M/1 -> Out22/1
  C2C_NMPC_constraints_up_IMEP/1 -> Out13/1
  C2C_NMPC_constraints_up_NOX/1 -> Out14/1
  C2C_NMPC_constraints_up_MPRR/1 -> Out16/1
  C2C_NMPC_constraints_up_SOOT/1 -> Out15/1
  C2C_NMPC_constraints_low_dt_SOI_main/1 -> Out19/1
  C2C_NMPC_constraints_low_dt_DOI_main/1 -> Out17/1
  C2C_NMPC_constraints_up_DOI_H2/1 -> Out8/1
  C2C_NMPC_constraints_up_dt_DOI_H1/1 -> Out24/1
  C2C_NMPC_constraints_up_dt_SOI_main/1 -> Out23/1
  C2C_NMPC_constraints_low_dt_P2M/1 -> Out18/1
  C2C_NMPC_constraints_low_dt_DOI_H2/1 -> Out20/1

== system sim_SS_H2DF_2024a_GRU/dynamics/C2C_NMPC/C2C_NMPC_n3/constraints1/Normalizing data ==
  physical_data : Inport
  Constant1 : Constant  Value=C2C_NMPC.Normalization.controls.mean(2)
  Constant2 : Constant  Value=C2C_NMPC.Normalization.controls.mean(3)
  Constant3 : Constant  Value=C2C_NMPC.Normalization.controls.mean(1)
  Constant4 : Constant  Value=C2C_NMPC.Normalization.controls.mean(4)
  Gain1 : Gain  Gain=1/C2C_NMPC.Normalization.controls.std(2)
  Gain2 : Gain  Gain=1/C2C_NMPC.Normalization.controls.std(3)
  Gain3 : Gain  Gain=1/C2C_NMPC.Normalization.controls.std(4)
  Gain4 : Gain  Gain=1/C2C_NMPC.Normalization.controls.std(1)
  Mux : Mux
  Selector : Selector  IndexOptions=Index vector (dialog)  Indices=[2]  OutputSizes=1
  Selector1 : Selector  IndexOptions=Index vector (dialog)  Indices=[1]  OutputSizes=1
  Selector2 : Selector  IndexOptions=Index vector (dialog)  Indices=[3]  OutputSizes=1
  Selector3 : Selector  IndexOptions=Index vector (dialog)  Indices=[4]  OutputSizes=1
  Sum{1..4} (4 alike) : Sum  Inputs=|+-
  normalized_data : Outport
  wires:
  Constant3/1 -> Sum4/2
  Selector2/1 -> Sum3/1
  Constant2/1 -> Sum3/2
  Sum4/1 -> Gain4/1
  Sum3/1 -> Gain2/1
  Selector/1 -> Sum2/1
  Constant1/1 -> Sum2/2
  Sum2/1 -> Gain1/1
  Sum1/1 -> Gain3/1
  Constant4/1 -> Sum1/2
  Selector3/1 -> Sum1/1
  Selector1/1 -> Sum4/1
  Gain4/1 -> Mux/1
  Gain1/1 -> Mux/2
  Gain2/1 -> Mux/3
  Gain3/1 -> Mux/4
  Mux/1 -> normalized_data/1
  physical_data/1 -> Selector1/1, Selector/1, Selector3/1, Selector2/1

== system sim_SS_H2DF_2024a_GRU/dynamics/C2C_NMPC/C2C_NMPC_n3/constraints1/Normalizing data Output ==
  In : Inport
  Constant : Constant  Value=C2C_NMPC.Normalization.outputs.mean(1)
  Constant1 : Constant  Value=C2C_NMPC.Normalization.outputs.mean(2)
  Constant2 : Constant  Value=C2C_NMPC.Normalization.outputs.mean(3)
  Constant3 : Constant  Value=C2C_NMPC.Normalization.outputs.mean(4)
  Demux : Demux
  Gain : Gain  Gain=1/C2C_NMPC.Normalization.outputs.std(1)
  Gain1 : Gain  Gain=1/C2C_NMPC.Normalization.outputs.std(2)
  Gain2 : Gain  Gain=1/C2C_NMPC.Normalization.outputs.std(3)
  Gain3 : Gain  Gain=1/C2C_NMPC.Normalization.outputs.std(4)
  Mux : Mux
  Sum{1..3,5} (4 alike) : Sum  Inputs=|+-
  value : Outport
  wires:
  Constant/1 -> Sum5/2
  Constant1/1 -> Sum1/2
  Sum1/1 -> Gain1/1
  Demux/3 -> Sum2/1
  Sum2/1 -> Gain2/1
  Constant2/1 -> Sum2/2
  Gain/1 -> Mux/1
  Sum3/1 -> Gain3/1
  Constant3/1 -> Sum3/2
  Sum5/1 -> Gain/1
  Demux/1 -> Sum5/1
  Gain2/1 -> Mux/3
  Gain3/1 -> Mux/4
  Gain1/1 -> Mux/2
  Demux/2 -> Sum1/1
  Demux/4 -> Sum3/1
  In/1 -> Demux/1
  Mux/1 -> value/1

== system sim_SS_H2DF_2024a_GRU/dynamics/C2C_NMPC/C2C_NMPC_n3/constraints1/Normalizing data1 ==
  physical_data : Inport
  Constant1 : Constant  Value=C2C_NMPC.Normalization.controls.mean(2)
  Constant2 : Constant  Value=C2C_NMPC.Normalization.controls.mean(3)
  Constant3 : Constant  Value=C2C_NMPC.Normalization.controls.mean(1)
  Constant4 : Constant  Value=C2C_NMPC.Normalization.controls.mean(4)
  Gain1 : Gain  Gain=1/C2C_NMPC.Normalization.controls.std(2)
  Gain2 : Gain  Gain=1/C2C_NMPC.Normalization.controls.std(3)
  Gain3 : Gain  Gain=1/C2C_NMPC.Normalization.controls.std(4)
  Gain4 : Gain  Gain=1/C2C_NMPC.Normalization.controls.std(1)
  Mux : Mux
  Selector : Selector  IndexOptions=Index vector (dialog)  Indices=[2]  OutputSizes=1
  Selector1 : Selector  IndexOptions=Index vector (dialog)  Indices=[1]  OutputSizes=1
  Selector2 : Selector  IndexOptions=Index vector (dialog)  Indices=[3]  OutputSizes=1
  Selector3 : Selector  IndexOptions=Index vector (dialog)  Indices=[4]  OutputSizes=1
  Sum{1..4} (4 alike) : Sum  Inputs=|+-
  normalized_data : Outport
  wires:
  Constant3/1 -> Sum4/2
  Selector2/1 -> Sum3/1
  Constant2/1 -> Sum3/2
  Sum4/1 -> Gain4/1
  Sum3/1 -> Gain2/1
  Selector/1 -> Sum2/1
  Constant1/1 -> Sum2/2
  Sum2/1 -> Gain1/1
  Sum1/1 -> Gain3/1
  Constant4/1 -> Sum1/2
  Selector3/1 -> Sum1/1
  Selector1/1 -> Sum4/1
  Gain4/1 -> Mux/1
  Gain1/1 -> Mux/2
  Gain2/1 -> Mux/3
  Gain3/1 -> Mux/4
  Mux/1 -> normalized_data/1
  physical_data/1 -> Selector1/1, Selector/1, Selector3/1, Selector2/1

== system sim_SS_H2DF_2024a_GRU/dynamics/C2C_NMPC/C2C_NMPC_n3/constraints1/Subsystem ==
  In : Inport
  Constant : Constant  Value=C2C_NMPC.Normalization.outputs.mean(1)
  Constant1 : Constant  Value=C2C_NMPC.Normalization.outputs.mean(2)
  Constant2 : Constant  Value=C2C_NMPC.Normalization.outputs.mean(3)
  Constant3 : Constant  Value=C2C_NMPC.Normalization.outputs.mean(4)
  Demux : Demux
  Gain : Gain  Gain=1/C2C_NMPC.Normalization.outputs.std(1)
  Gain1 : Gain  Gain=1/C2C_NMPC.Normalization.outputs.std(2)
  Gain2 : Gain  Gain=1/C2C_NMPC.Normalization.outputs.std(3)
  Gain3 : Gain  Gain=1/C2C_NMPC.Normalization.outputs.std(4)
  Mux : Mux
  Sum{1..3,5} (4 alike) : Sum  Inputs=|+-
  value : Outport
  wires:
  Constant/1 -> Sum5/2
  Constant1/1 -> Sum1/2
  Sum1/1 -> Gain1/1
  Demux/3 -> Sum2/1
  Sum2/1 -> Gain2/1
  Constant2/1 -> Sum2/2
  Gain/1 -> Mux/1
  Sum3/1 -> Gain3/1
  Constant3/1 -> Sum3/2
  Sum5/1 -> Gain/1
  Demux/1 -> Sum5/1
  Gain2/1 -> Mux/3
  Gain3/1 -> Mux/4
  Gain1/1 -> Mux/2
  Demux/2 -> Sum1/1
  Demux/4 -> Sum3/1
  In/1 -> Demux/1
  Mux/1 -> value/1

== system sim_SS_H2DF_2024a_GRU/dynamics/C2C_NMPC/C2C_NMPC_n3/constraints1/Subsystem1 ==
  In : Inport
  Constant : Constant  Value=C2C_NMPC.Normalization.outputs.mean(1)
  Constant1 : Constant  Value=C2C_NMPC.Normalization.outputs.mean(2)
  Constant2 : Constant  Value=C2C_NMPC.Normalization.outputs.mean(3)
  Constant3 : Constant  Value=C2C_NMPC.Normalization.outputs.mean(4)
  Demux : Demux
  Gain : Gain  Gain=1/C2C_NMPC.Normalization.outputs.std(1)
  Gain1 : Gain  Gain=1/C2C_NMPC.Normalization.outputs.std(2)
  Gain2 : Gain  Gain=1/C2C_NMPC.Normalization.outputs.std(3)
  Gain3 : Gain  Gain=1/C2C_NMPC.Normalization.outputs.std(4)
  Mux : Mux
  Sum{1..3,5} (4 alike) : Sum  Inputs=|+-
  ubh_e : Outport
  wires:
  Mux/1 -> ubh_e/1
  In/1 -> Demux/1
  Demux/4 -> Sum3/1
  Demux/2 -> Sum1/1
  Gain1/1 -> Mux/2
  Gain3/1 -> Mux/4
  Gain2/1 -> Mux/3
  Demux/1 -> Sum5/1
  Sum5/1 -> Gain/1
  Constant3/1 -> Sum3/2
  Sum3/1 -> Gain3/1
  Gain/1 -> Mux/1
  Constant2/1 -> Sum2/2
  Sum2/1 -> Gain2/1
  Demux/3 -> Sum2/1
  Sum1/1 -> Gain1/1
  Constant1/1 -> Sum1/2
  Constant/1 -> Sum5/2

== system sim_SS_H2DF_2024a_GRU/dynamics/C2C_NMPC/C2C_NMPC_n3/constraints1/Subsystem2 ==
  In : Inport
  Demux : Demux
  Gain : Gain  Gain=1/C2C_NMPC.Normalization.controls.std(1)
  Gain1 : Gain  Gain=1/C2C_NMPC.Normalization.controls.std(2)
  Gain2 : Gain  Gain=1/C2C_NMPC.Normalization.controls.std(3)
  Gain3 : Gain  Gain=1/C2C_NMPC.Normalization.controls.std(4)
  Mux : Mux
  Out : Outport
  wires:
  Gain/1 -> Mux/1
  Gain2/1 -> Mux/3
  Gain1/1 -> Mux/2
  In/1 -> Demux/1
  Mux/1 -> Out/1
  Demux/1 -> Gain/1
  Demux/2 -> Gain1/1
  Demux/3 -> Gain2/1
  Demux/4 -> Gain3/1
  Gain3/1 -> Mux/4

== system sim_SS_H2DF_2024a_GRU/dynamics/C2C_NMPC/C2C_NMPC_n3/constraints1/Subsystem3 ==
  In : Inport
  Demux : Demux
  Gain : Gain  Gain=1/C2C_NMPC.Normalization.controls.std(1)
  Gain1 : Gain  Gain=1/C2C_NMPC.Normalization.controls.std(2)
  Gain2 : Gain  Gain=1/C2C_NMPC.Normalization.controls.std(3)
  Gain3 : Gain  Gain=1/C2C_NMPC.Normalization.controls.std(4)
  Mux : Mux
  Out : Outport
  wires:
  Gain/1 -> Mux/1
  Gain2/1 -> Mux/3
  Gain1/1 -> Mux/2
  In/1 -> Demux/1
  Mux/1 -> Out/1
  Demux/1 -> Gain/1
  Demux/2 -> Gain1/1
  Demux/3 -> Gain2/1
  Demux/4 -> Gain3/1
  Gain3/1 -> Mux/4

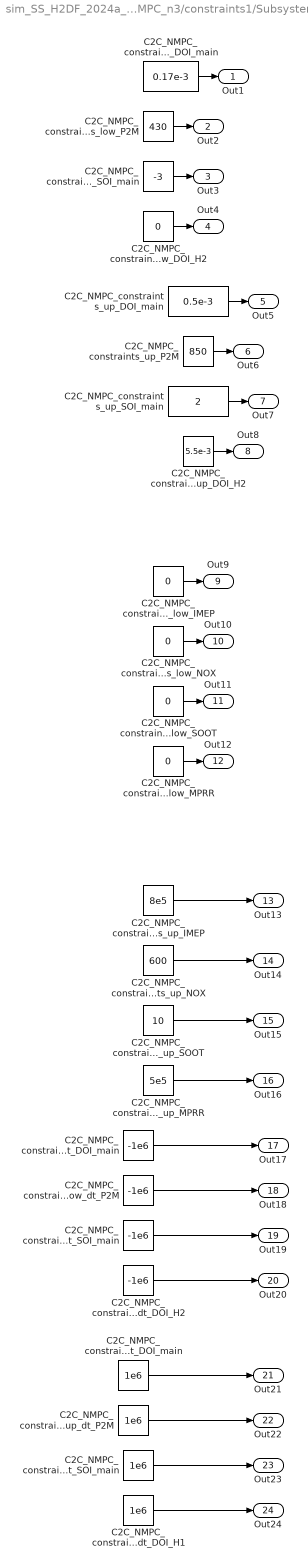
== system sim_SS_H2DF_2024a_GRU/dynamics/C2C_NMPC/C2C_NMPC_n3/constraints1/Subsystem4 ==
  C2C_NMPC_constraints_low_DOI_H2 : Constant  Value=0
  C2C_NMPC_constraints_low_DOI_main : Constant  Value=0.17e-3
  C2C_NMPC_constraints_low_IMEP : Constant  Value=0
  C2C_NMPC_constraints_low_MPRR : Constant  Value=0
  C2C_NMPC_constraints_low_NOX : Constant  Value=0
  C2C_NMPC_constraints_low_P2M : Constant  Value=430
  C2C_NMPC_constraints_low_SOI_main : Constant  Value=-3
  C2C_NMPC_constraints_low_SOOT : Constant  Value=0
  C2C_NMPC_constraints_low_dt_DOI_H2 : Constant  Value=-1e6
  C2C_NMPC_constraints_low_dt_DOI_main : Constant  Value=-1e6
  C2C_NMPC_constraints_low_dt_P2M : Constant  Value=-1e6
  C2C_NMPC_constraints_low_dt_SOI_main : Constant  Value=-1e6
  C2C_NMPC_constraints_up_DOI_H2 : Constant  Value=5.5e-3
  C2C_NMPC_constraints_up_DOI_main : Constant  Value=0.5e-3
  C2C_NMPC_constraints_up_IMEP : Constant  Value=8e5
  C2C_NMPC_constraints_up_MPRR : Constant  Value=5e5
  C2C_NMPC_constraints_up_NOX : Constant  Value=600
  C2C_NMPC_constraints_up_P2M : Constant  Value=850
  C2C_NMPC_constraints_up_SOI_main : Constant  Value=2
  C2C_NMPC_constraints_up_SOOT : Constant  Value=10
  C2C_NMPC_constraints_up_dt_DOI_H1 : Constant  Value=1e6
  C2C_NMPC_constraints_up_dt_DOI_main : Constant  Value=1e6
  C2C_NMPC_constraints_up_dt_P2M : Constant  Value=1e6
  C2C_NMPC_constraints_up_dt_SOI_main : Constant  Value=1e6
  Out1 : Outport
  Out2 : Outport  Port=2
  Out3 : Outport  Port=3
  Out4 : Outport  Port=4
  Out5 : Outport  Port=5
  Out6 : Outport  Port=6
  Out7 : Outport  Port=7
  Out8 : Outport  Port=8
  Out9 : Outport  Port=9
  Out10 : Outport  Port=10
  Out11 : Outport  Port=11
  Out12 : Outport  Port=12
  Out13 : Outport  Port=13
  Out14 : Outport  Port=14
  Out15 : Outport  Port=15
  Out16 : Outport  Port=16
  Out17 : Outport  Port=17
  Out18 : Outport  Port=18
  Out19 : Outport  Port=19
  Out20 : Outport  Port=20
  Out21 : Outport  Port=21
  Out22 : Outport  Port=22
  Out23 : Outport  Port=23
  Out24 : Outport  Port=24
  wires:
  C2C_NMPC_constraints_low_dt_DOI_H2/1 -> Out20/1
  C2C_NMPC_constraints_low_dt_P2M/1 -> Out18/1
  C2C_NMPC_constraints_up_dt_SOI_main/1 -> Out23/1
  C2C_NMPC_constraints_up_dt_DOI_H1/1 -> Out24/1
  C2C_NMPC_constraints_up_DOI_H2/1 -> Out8/1
  C2C_NMPC_constraints_low_dt_DOI_main/1 -> Out17/1
  C2C_NMPC_constraints_low_dt_SOI_main/1 -> Out19/1
  C2C_NMPC_constraints_up_SOOT/1 -> Out15/1
  C2C_NMPC_constraints_up_MPRR/1 -> Out16/1
  C2C_NMPC_constraints_up_NOX/1 -> Out14/1
  C2C_NMPC_constraints_up_IMEP/1 -> Out13/1
  C2C_NMPC_constraints_up_dt_P2M/1 -> Out22/1
  C2C_NMPC_constraints_low_SOI_main/1 -> Out3/1
  C2C_NMPC_constraints_up_dt_DOI_main/1 -> Out21/1
  C2C_NMPC_constraints_low_SOOT/1 -> Out11/1
  C2C_NMPC_constraints_low_DOI_H2/1 -> Out4/1
  C2C_NMPC_constraints_up_P2M/1 -> Out6/1
  C2C_NMPC_constraints_low_P2M/1 -> Out2/1
  C2C_NMPC_constraints_low_DOI_main/1 -> Out1/1
  C2C_NMPC_constraints_low_MPRR/1 -> Out12/1
  C2C_NMPC_constraints_up_SOI_main/1 -> Out7/1
  C2C_NMPC_constraints_up_DOI_main/1 -> Out5/1
  C2C_NMPC_constraints_low_IMEP/1 -> Out9/1
  C2C_NMPC_constraints_low_NOX/1 -> Out10/1

== system sim_SS_H2DF_2024a_GRU/dynamics/C2C_NMPC/C2C_NMPC_n3/constraints1/Subsystem5 ==
  In : Inport
  Constant : Constant  Value=C2C_NMPC.Normalization.outputs.mean(1)
  Constant1 : Constant  Value=C2C_NMPC.Normalization.outputs.mean(2)
  Constant2 : Constant  Value=C2C_NMPC.Normalization.outputs.mean(3)
  Constant3 : Constant  Value=C2C_NMPC.Normalization.outputs.mean(4)
  Demux : Demux
  Gain : Gain  Gain=1/C2C_NMPC.Normalization.outputs.std(1)
  Gain1 : Gain  Gain=1/C2C_NMPC.Normalization.outputs.std(2)
  Gain2 : Gain  Gain=1/C2C_NMPC.Normalization.outputs.std(3)
  Gain3 : Gain  Gain=1/C2C_NMPC.Normalization.outputs.std(4)
  Mux : Mux
  Sum{1..3,5} (4 alike) : Sum  Inputs=|+-
  ubh_e : Outport
  wires:
  Mux/1 -> ubh_e/1
  In/1 -> Demux/1
  Demux/4 -> Sum3/1
  Demux/2 -> Sum1/1
  Gain1/1 -> Mux/2
  Gain3/1 -> Mux/4
  Gain2/1 -> Mux/3
  Demux/1 -> Sum5/1
  Sum5/1 -> Gain/1
  Constant3/1 -> Sum3/2
  Sum3/1 -> Gain3/1
  Gain/1 -> Mux/1
  Constant2/1 -> Sum2/2
  Sum2/1 -> Gain2/1
  Demux/3 -> Sum2/1
  Sum1/1 -> Gain1/1
  Constant1/1 -> Sum1/2
  Constant/1 -> Sum5/2

== matlab function sim_SS_H2DF_2024a_GRU/dynamics/C2C_NMPC/C2C_NMPC_n3/cost_function_weights/blkdiag Function ==
  data: u1 input; y output; u2 input; u3 input
 function y = fcn(u1,u2,u3)
y = reshape(blkdiag(u1, u2, u3),[],1);

== matlab function sim_SS_H2DF_2024a_GRU/dynamics/C2C_NMPC/C2C_NMPC_n3/cost_function_weights/blkdiag Function1 ==
  data: u1 input; y output; u2 input
function y = fcn(u1,u2)
y = reshape(blkdiag(u1, u2),[],1);

== matlab function sim_SS_H2DF_2024a_GRU/reference/reference_dynamic/reference_dynamic/ref_func ==
  data: ref_norm input; y_ref output size=horizon_length * cost_length; init_index input size=1; y_ref_buf parameter; cost_length parameter size=1; horizon_length parameter size=1
function y_ref = ref_func(ref_norm, init_index, y_ref_buf, cost_length, horizon_length)
% more init in callbacks

% init output
y_ref = zeros(cost_length*horizon_length, 1);

if init_index == 4899
    y_ref_buf(:, 1) = ref_norm(:, init_index);
    y_ref_buf(:, 2) = ref_norm(:, init_index+1);
    y_ref_buf(:, 3) = ref_norm(:, init_index+1);
elseif init_index == 4900
    y_ref_buf(:, 1) = ref_norm(:, init_index);
    y_ref_buf(:, 2) = ref_norm(:, init_index);
    y_ref_buf(:, 3) = ref_norm(:, init_index);
else
    y_ref_buf(:, 1) = ref_norm(:, init_index);
    y_ref_buf(:, 2) = ref_norm(:, init_index+1);
    y_ref_buf(:, 3) = ref_norm(:, init_index+2); 
end

y_ref(1:cost_length) = y_ref_buf(:,1);
y_ref( (cost_length+1) : (cost_length * 2) ) = y_ref_buf(:,2);
y_ref( ((cost_length*2)+1) : (cost_length * 3) ) = y_ref_buf(:,3);

== matlab function sim_SS_H2DF_2024a_GRU/dynamics/C2C_NMPC/C2C_NMPC_n3/constraints1/MATLAB Function ==
  data: value input; vector output; length input; init_vector input
function vector = fcn(value, length, init_vector)
init_vector(1:(size(value,1)*length)) = repmat(value, length, 1);
vector = init_vector;

== matlab function sim_SS_H2DF_2024a_GRU/dynamics/C2C_NMPC/C2C_NMPC_n3/constraints1/MATLAB Function1 ==
  data: value input; vector output; length input; init_vector input
function vector = fcn(value, length, init_vector)
init_vector(1:(size(value,1)*length)) = repmat(value, length, 1);
vector = init_vector;

== matlab function sim_SS_H2DF_2024a_GRU/dynamics/C2C_NMPC/C2C_NMPC_n3/constraints1/MATLAB Function2 ==
  data: value input; vector output; length input; init_vector input
function vector = fcn(value, length, init_vector)
init_vector(1:(size(value,1)*length)) = repmat(value, length, 1);
vector = init_vector;

== matlab function sim_SS_H2DF_2024a_GRU/dynamics/C2C_NMPC/C2C_NMPC_n3/constraints1/MATLAB Function3 ==
  data: value input; vector output; length input; init_vector input
function vector = fcn(value, length, init_vector)
init_vector(1:(size(value,1)*length)) = repmat(value, length, 1);
vector = init_vector;

== matlab function sim_SS_H2DF_2024a_GRU/dynamics/C2C_NMPC/C2C_NMPC_n3/constraints1/MATLAB Function4 ==
  data: value input; vector output; length input; init_vector input
function vector = fcn(value, length, init_vector)
init_vector(1:(size(value,1)*length)) = repmat(value, length, 1);
vector = init_vector;

== matlab function sim_SS_H2DF_2024a_GRU/dynamics/C2C_NMPC/C2C_NMPC_n3/constraints1/MATLAB Function5 ==
  data: value input; vector output; length input; init_vector input
function vector = fcn(value, length, init_vector)
init_vector(1:(size(value,1)*length)) = repmat(value, length, 1);
vector = init_vector;

== matlab function sim_SS_H2DF_2024a_GRU/dynamics/dyn_H2DF/dyn_H2DF/dyn_H2DF ==
  data: last_LSTM_states input; controls input; last_outputs input; outputs output; H2DF_Par parameter; LSTM_states output
function [outputs, LSTM_states] = dyn_H2DF(last_LSTM_states, controls, last_outputs, H2DF_Par)

[outputs, LSTM_states] = dyn_H2DF_GRU(last_LSTM_states, [controls; last_outputs(1)], H2DF_Par);

== matlab function sim_SS_H2DF_2024a_GRU/dynamics/dyn_H2DF_state_augmentation/dyn_H2DF_state_augmentation_nofb/dyn_H2DF_state_augmentation ==
  data: last_LSTM_states input; LSTM_states output; controls input; H2DF_Par parameter
function LSTM_states = dyn_H2DF_state_augmentation(last_LSTM_states, controls, H2DF_Par)

LSTM_states = dyn_H2DF_state_augmentation_GRU(last_LSTM_states,controls, H2DF_Par);

== matlab function sim_SS_H2DF_2024a_GRU/dynamics/dyn_H2DF/dyn_H2DF_nofb/dyn_H2DF ==
  data: last_LSTM_states input; controls input; outputs output; H2DF_Par parameter; LSTM_states output
function [outputs, LSTM_states] = dyn_H2DF(last_LSTM_states, controls, H2DF_Par)

[outputs, LSTM_states] = dyn_H2DF_GRU(last_LSTM_states, controls, H2DF_Par);

== matlab function sim_SS_H2DF_2024a_GRU/reference/reference_static/ref_func ==
  data: ref_norm input; y_ref output; init_index input
function y_ref = ref_func(ref_norm, init_index)

y_ref = ref_norm(:, init_index);

== matlab function sim_SS_H2DF_2024a_GRU/dynamics/C2C_NMPC/C2C_NMPC_n3/constraints (no soft)/MATLAB Function ==
  data: value input; vector output; length input; init_vector input
function vector = fcn(value, length, init_vector)
init_vector(1:(size(value,1)*length)) = repmat(value, length, 1);
vector = init_vector;

== matlab function sim_SS_H2DF_2024a_GRU/dynamics/dyn_H2DF_state_augmentation/dyn_H2DF_state_augmentation/dyn_H2DF_state_augmentation ==
  data: last_LSTM_states input; LSTM_states output; controls input; last_outputs input; H2DF_Par parameter
function LSTM_states = dyn_H2DF_state_augmentation(last_LSTM_states, controls, last_outputs, H2DF_Par)

LSTM_states = dyn_H2DF_state_augmentation_GRU(last_LSTM_states,[controls; last_outputs(1)], H2DF_Par);

== matlab function sim_SS_H2DF_2024a_GRU/dynamics/C2C_NMPC/C2C_NMPC_n3/constraints (no soft)/MATLAB Function1 ==
  data: value input; vector output; length input; init_vector input
function vector = fcn(value, length, init_vector)
init_vector(1:(size(value,1)*length)) = repmat(value, length, 1);
vector = init_vector;
